simulink model "smMarsRover"  (R2024b)
settings: Solver=VariableStepAuto  StartTime=0.0  StopTime=51  RelTol=1e-3
PreLoadFcn:
  | run_sm
values from neighbouring files (symbols this model uses):
  arm_q0 = [-2.3554 -125.9144   49.8193 -175.7336  177.6446  180.0000]    [sm_mars_rover_params.m]
  goal_loc = [roverPath.x(end) roverPath.y(end)]    [sm_mars_rover_params.m]
  Z = fillmissing(Z, 'linear')    [setup.m]
undefined symbols (not defined in the file or in its folder): cameraData, Chassis_L, Chassis_width, eeConfig, Kd, Kd_arm, Kd_steer, Ki, Ki_arm, Ki_steer, Kp, Kp_arm, Kp_steer, Link1, Link2, Link3, R_disc_Link1, rover_accel, roverPath, t1, TrqLoLimit, TrqUpLimit, Wheel1_G, Wheel2_G, Wheel3_G, Wheel4_G, Wheel5_G, Wheel6_G, Wheel_Radius, X, Y
libraries: sm_lib x216, nesl_utility x51, slpidlib x3, simulink x3, robotcorelib x1, robotalgslib x1, simulink_extras x1
(part 7 of 7)

== system smMarsRover/RoverMotionControl&Planning/Rover /Wheels/RBWheel ==
  InnerWheel : sm_lib/Body Elements/File Solid  ExtGeomFileName=sm_mars_RoverData\mobility_wheel_inner.stl  UnitType=Custom  ExtGeomFileUnits=cm  StepReaderType=HEX  ExportConvexHullGeometry=off  InertiaType=Custom  BasedOnType=Density  Density=1000  DensityUnits=kg/m^3  Mass=0  MassUnits=kg  CenterOfMass=[0 0 0]  CenterOfMassUnits=m  MomentsOfInertia=[1 1 1]*0  MomentsOfInertiaUnits=kg*m^2  ProductsOfInertia=[0 0 0]  ProductsOfInertiaUnits=kg*m^2  GraphicType=FromGeometry  MarkerShape=Sphere  MarkerSize=10  GraphicVisPropType=AdvancedVisualProperties  GraphicDiffuseColor=[1.0 1.0 1.0]  GraphicOpacity=1.0  GraphicSpecularColor=[1 1 1 1.0]  GraphicAmbientColor=[0.15 0.15 0.15 1.0]  GraphicEmissiveColor=[0.1 0.1 0 1.0]  GraphicShininess=90  DoExposeReferenceFrame=on  SerializedFrames=<Frames/>
  OuterWheel : sm_lib/Body Elements/File Solid  ExtGeomFileName=sm_mars_RoverData\mobility_wheel_outer.stl  UnitType=Custom  ExtGeomFileUnits=cm  StepReaderType=HEX  ExportConvexHullGeometry=off  InertiaType=CalculateFromGeometry  BasedOnType=Density  Density=2700  DensityUnits=kg/m^3  Mass=1  MassUnits=kg  CenterOfMass=[0 0 0]  CenterOfMassUnits=m  MomentsOfInertia=[1 1 1]  MomentsOfInertiaUnits=kg*m^2  ProductsOfInertia=[0 0 0]  ProductsOfInertiaUnits=kg*m^2  GraphicType=FromGeometry  MarkerShape=Sphere  MarkerSize=10  GraphicVisPropType=AdvancedVisualProperties  GraphicDiffuseColor=[0.15 0.15 0.15]  GraphicOpacity=1.0  GraphicSpecularColor=[1 1 1 1.0]  GraphicAmbientColor=[0.15 0.15 0.15 1.0]  GraphicEmissiveColor=[0. 0. 0. 1]  GraphicShininess=100  DoExposeReferenceFrame=on  SerializedFrames=<Frames/>
  Point Cloud : sm_lib/Curves and Surfaces/Point Cloud  CoordinatesMatrix=new_wheel_points  CoordinatesMatrixUnits=cm  GraphicType=MarkerCloud  GraphicSphereRadius=0.25  GraphicSphereRadiusUnits=cm  GraphicVisPropType=SimpleVisualProperties  GraphicDiffuseColor=[1 0 0]  GraphicOpacity=1.0  GraphicSpecularColor=[0.5 0.5 0.5 1.0]  GraphicAmbientColor=[0.15 0.15 0.15 1.0]  GraphicEmissiveColor=[0.0 0.0 0.0 1.0]  GraphicShininess=75
  Rigid Transform : sm_lib/Frames and Transforms/Rigid Transform  RotationMethod=RotationMatrix  FollAlignAxisA=+X  BaseAlignAxisA=+Y  FollAlignAxisB=+Y  BaseAlignAxisB=+Z  RotationStandardAxis=+Z  RotationAngle=0.0  RotationAngleUnits=deg  RotationArbitraryAxis=[0 0 1]  RotationSequenceAxes=FollowerAxes  RotationSequence=XYX  RotationSequenceAngles=[0 0 0]  RotationSequenceAnglesUnits=deg  RotationMatrix=Wheel.WRJ_R  Quaternion=[1 0 0 0]  TranslationMethod=Cartesian  TranslationCartesianOffset=Wheel.WRJ_T  TranslationCartesianOffsetUnits=m  TranslationStandardAxis=+Z  TranslationStandardOffset=0  TranslationStandardOffsetUnits=m  TranslationROffset=0  TranslationROffsetUnits=m  TranslationThetaOffset=0  TranslationThetaOffsetUnits=deg  TranslationZOffset=0  TranslationZOffsetUnits=m
  Rigid Transform6 : sm_lib/Frames and Transforms/Rigid Transform  RotationMethod=StandardAxis  FollAlignAxisA=+X  BaseAlignAxisA=+Y  FollAlignAxisB=+Y  BaseAlignAxisB=+Z  RotationStandardAxis=+X  RotationAngle=90  RotationAngleUnits=deg  RotationArbitraryAxis=[0 0 1]  RotationSequenceAxes=FollowerAxes  RotationSequence=XYX  RotationSequenceAngles=[0 0 0]  RotationSequenceAnglesUnits=deg  RotationMatrix=[1 0 0; 0 1 0; 0 0 1]  Quaternion=[1 0 0 0]  TranslationMethod=None  TranslationCartesianOffset=[0 0 0]  TranslationCartesianOffsetUnits=cm  TranslationStandardAxis=+Y  TranslationStandardOffset=25.500/2  TranslationStandardOffsetUnits=cm  TranslationROffset=0  TranslationROffsetUnits=m  TranslationThetaOffset=0  TranslationThetaOffsetUnits=deg  TranslationZOffset=0  TranslationZOffsetUnits=m
  WRJ : PMIOPort  Side=Right
  G : PMIOPort  Port=2  Side=Left
  connections:
  Rigid Transform6/RConn1 -- WRJ/RConn1 -- Rigid Transform/RConn1
  OuterWheel/RConn1 -- Point Cloud/LConn1 -- Rigid Transform6/LConn1
  G/RConn1 -- Point Cloud/RConn1
  InnerWheel/RConn1 -- Rigid Transform/LConn1

== system smMarsRover/RoverMotionControl&Planning/Rover /Wheels/RFWheel ==
  InnerWheel : sm_lib/Body Elements/File Solid  ExtGeomFileName=sm_mars_RoverData\mobility_wheel_inner.stl  UnitType=Custom  ExtGeomFileUnits=cm  StepReaderType=HEX  ExportConvexHullGeometry=off  InertiaType=Custom  BasedOnType=Density  Density=1000  DensityUnits=kg/m^3  Mass=0  MassUnits=kg  CenterOfMass=[0 0 0]  CenterOfMassUnits=m  MomentsOfInertia=[1 1 1]*0  MomentsOfInertiaUnits=kg*m^2  ProductsOfInertia=[0 0 0]  ProductsOfInertiaUnits=kg*m^2  GraphicType=FromGeometry  MarkerShape=Sphere  MarkerSize=10  GraphicVisPropType=AdvancedVisualProperties  GraphicDiffuseColor=[1.0 1.0 1.0]  GraphicOpacity=1.0  GraphicSpecularColor=[1 1 1 1.0]  GraphicAmbientColor=[0.15 0.15 0.15 1.0]  GraphicEmissiveColor=[0.1 0.1 0 1.0]  GraphicShininess=90  DoExposeReferenceFrame=on  SerializedFrames=<Frames/>
  OuterWheel : sm_lib/Body Elements/File Solid  ExtGeomFileName=sm_mars_RoverData\mobility_wheel_outer.stl  UnitType=Custom  ExtGeomFileUnits=cm  StepReaderType=HEX  ExportConvexHullGeometry=off  InertiaType=CalculateFromGeometry  BasedOnType=Density  Density=2700  DensityUnits=kg/m^3  Mass=1  MassUnits=kg  CenterOfMass=[0 0 0]  CenterOfMassUnits=m  MomentsOfInertia=[1 1 1]  MomentsOfInertiaUnits=kg*m^2  ProductsOfInertia=[0 0 0]  ProductsOfInertiaUnits=kg*m^2  GraphicType=FromGeometry  MarkerShape=Sphere  MarkerSize=10  GraphicVisPropType=AdvancedVisualProperties  GraphicDiffuseColor=[0.15 0.15 0.15]  GraphicOpacity=1.0  GraphicSpecularColor=[1 1 1 1.0]  GraphicAmbientColor=[0.15 0.15 0.15 1.0]  GraphicEmissiveColor=[0. 0. 0. 1]  GraphicShininess=100  DoExposeReferenceFrame=on  SerializedFrames=<Frames/>
  Point Cloud : sm_lib/Curves and Surfaces/Point Cloud  CoordinatesMatrix=new_wheel_points  CoordinatesMatrixUnits=cm  GraphicType=MarkerCloud  GraphicSphereRadius=0.25  GraphicSphereRadiusUnits=cm  GraphicVisPropType=SimpleVisualProperties  GraphicDiffuseColor=[1 0 0]  GraphicOpacity=1.0  GraphicSpecularColor=[0.5 0.5 0.5 1.0]  GraphicAmbientColor=[0.15 0.15 0.15 1.0]  GraphicEmissiveColor=[0.0 0.0 0.0 1.0]  GraphicShininess=75
  Rigid Transform : sm_lib/Frames and Transforms/Rigid Transform  RotationMethod=RotationMatrix  FollAlignAxisA=+X  BaseAlignAxisA=+Y  FollAlignAxisB=+Y  BaseAlignAxisB=+Z  RotationStandardAxis=+Z  RotationAngle=0.0  RotationAngleUnits=deg  RotationArbitraryAxis=[0 0 1]  RotationSequenceAxes=FollowerAxes  RotationSequence=XYX  RotationSequenceAngles=[0 0 0]  RotationSequenceAnglesUnits=deg  RotationMatrix=Wheel.WRJ_R  Quaternion=[1 0 0 0]  TranslationMethod=Cartesian  TranslationCartesianOffset=Wheel.WRJ_T  TranslationCartesianOffsetUnits=m  TranslationStandardAxis=+Z  TranslationStandardOffset=0  TranslationStandardOffsetUnits=m  TranslationROffset=0  TranslationROffsetUnits=m  TranslationThetaOffset=0  TranslationThetaOffsetUnits=deg  TranslationZOffset=0  TranslationZOffsetUnits=m
  Rigid Transform6 : sm_lib/Frames and Transforms/Rigid Transform  RotationMethod=StandardAxis  FollAlignAxisA=+X  BaseAlignAxisA=+Y  FollAlignAxisB=+Y  BaseAlignAxisB=+Z  RotationStandardAxis=+X  RotationAngle=90  RotationAngleUnits=deg  RotationArbitraryAxis=[0 0 1]  RotationSequenceAxes=FollowerAxes  RotationSequence=XYX  RotationSequenceAngles=[0 0 0]  RotationSequenceAnglesUnits=deg  RotationMatrix=[1 0 0; 0 1 0; 0 0 1]  Quaternion=[1 0 0 0]  TranslationMethod=None  TranslationCartesianOffset=[0 0 0]  TranslationCartesianOffsetUnits=cm  TranslationStandardAxis=+Y  TranslationStandardOffset=25.500/2  TranslationStandardOffsetUnits=cm  TranslationROffset=0  TranslationROffsetUnits=m  TranslationThetaOffset=0  TranslationThetaOffsetUnits=deg  TranslationZOffset=0  TranslationZOffsetUnits=m
  WRJ : PMIOPort  Side=Right
  G : PMIOPort  Port=2  Side=Left
  connections:
  InnerWheel/RConn1 -- Rigid Transform/LConn1
  G/RConn1 -- Point Cloud/RConn1
  Rigid Transform6/LConn1 -- Point Cloud/LConn1 -- OuterWheel/RConn1
  Rigid Transform/RConn1 -- WRJ/RConn1 -- Rigid Transform6/RConn1

== system smMarsRover/RoverMotionControl&Planning/Rover /Wheels/RMWheel ==
  InnerWheel : sm_lib/Body Elements/File Solid  ExtGeomFileName=sm_mars_RoverData\mobility_wheel_inner.stl  UnitType=Custom  ExtGeomFileUnits=cm  StepReaderType=HEX  ExportConvexHullGeometry=off  InertiaType=Custom  BasedOnType=Density  Density=1000  DensityUnits=kg/m^3  Mass=0  MassUnits=kg  CenterOfMass=[0 0 0]  CenterOfMassUnits=m  MomentsOfInertia=[1 1 1]*0  MomentsOfInertiaUnits=kg*m^2  ProductsOfInertia=[0 0 0]  ProductsOfInertiaUnits=kg*m^2  GraphicType=FromGeometry  MarkerShape=Sphere  MarkerSize=10  GraphicVisPropType=AdvancedVisualProperties  GraphicDiffuseColor=[1.0 1.0 1.0]  GraphicOpacity=1.0  GraphicSpecularColor=[1 1 1 1.0]  GraphicAmbientColor=[0.15 0.15 0.15 1.0]  GraphicEmissiveColor=[0.1 0.1 0 1.0]  GraphicShininess=90  DoExposeReferenceFrame=on  SerializedFrames=<Frames/>
  OuterWheel : sm_lib/Body Elements/File Solid  ExtGeomFileName=sm_mars_RoverData\mobility_wheel_outer.stl  UnitType=Custom  ExtGeomFileUnits=cm  StepReaderType=HEX  ExportConvexHullGeometry=off  InertiaType=CalculateFromGeometry  BasedOnType=Density  Density=2700  DensityUnits=kg/m^3  Mass=1  MassUnits=kg  CenterOfMass=[0 0 0]  CenterOfMassUnits=m  MomentsOfInertia=[1 1 1]  MomentsOfInertiaUnits=kg*m^2  ProductsOfInertia=[0 0 0]  ProductsOfInertiaUnits=kg*m^2  GraphicType=FromGeometry  MarkerShape=Sphere  MarkerSize=10  GraphicVisPropType=AdvancedVisualProperties  GraphicDiffuseColor=[0.15 0.15 0.15]  GraphicOpacity=1.0  GraphicSpecularColor=[1 1 1 1.0]  GraphicAmbientColor=[0.15 0.15 0.15 1.0]  GraphicEmissiveColor=[0. 0. 0. 1]  GraphicShininess=100  DoExposeReferenceFrame=on  SerializedFrames=<Frames/>
  Point Cloud : sm_lib/Curves and Surfaces/Point Cloud  CoordinatesMatrix=new_wheel_points  CoordinatesMatrixUnits=cm  GraphicType=MarkerCloud  GraphicSphereRadius=0.25  GraphicSphereRadiusUnits=cm  GraphicVisPropType=SimpleVisualProperties  GraphicDiffuseColor=[1 0 0]  GraphicOpacity=1.0  GraphicSpecularColor=[0.5 0.5 0.5 1.0]  GraphicAmbientColor=[0.15 0.15 0.15 1.0]  GraphicEmissiveColor=[0.0 0.0 0.0 1.0]  GraphicShininess=75
  Rigid Transform : sm_lib/Frames and Transforms/Rigid Transform  RotationMethod=RotationMatrix  FollAlignAxisA=+X  BaseAlignAxisA=+Y  FollAlignAxisB=+Y  BaseAlignAxisB=+Z  RotationStandardAxis=+Z  RotationAngle=0.0  RotationAngleUnits=deg  RotationArbitraryAxis=[0 0 1]  RotationSequenceAxes=FollowerAxes  RotationSequence=XYX  RotationSequenceAngles=[0 0 0]  RotationSequenceAnglesUnits=deg  RotationMatrix=Wheel.WRJ_R  Quaternion=[1 0 0 0]  TranslationMethod=Cartesian  TranslationCartesianOffset=Wheel.WRJ_T  TranslationCartesianOffsetUnits=m  TranslationStandardAxis=+Z  TranslationStandardOffset=0  TranslationStandardOffsetUnits=m  TranslationROffset=0  TranslationROffsetUnits=m  TranslationThetaOffset=0  TranslationThetaOffsetUnits=deg  TranslationZOffset=0  TranslationZOffsetUnits=m
  Rigid Transform6 : sm_lib/Frames and Transforms/Rigid Transform  RotationMethod=StandardAxis  FollAlignAxisA=+X  BaseAlignAxisA=+Y  FollAlignAxisB=+Y  BaseAlignAxisB=+Z  RotationStandardAxis=+X  RotationAngle=90  RotationAngleUnits=deg  RotationArbitraryAxis=[0 0 1]  RotationSequenceAxes=FollowerAxes  RotationSequence=XYX  RotationSequenceAngles=[0 0 0]  RotationSequenceAnglesUnits=deg  RotationMatrix=[1 0 0; 0 1 0; 0 0 1]  Quaternion=[1 0 0 0]  TranslationMethod=None  TranslationCartesianOffset=[0 0 0]  TranslationCartesianOffsetUnits=cm  TranslationStandardAxis=+Y  TranslationStandardOffset=25.500/2  TranslationStandardOffsetUnits=cm  TranslationROffset=0  TranslationROffsetUnits=m  TranslationThetaOffset=0  TranslationThetaOffsetUnits=deg  TranslationZOffset=0  TranslationZOffsetUnits=m
  WRJ : PMIOPort  Side=Right
  G : PMIOPort  Port=2  Side=Left
  connections:
  InnerWheel/RConn1 -- Rigid Transform/LConn1
  G/RConn1 -- Point Cloud/RConn1
  Rigid Transform6/LConn1 -- Point Cloud/LConn1 -- OuterWheel/RConn1
  Rigid Transform/RConn1 -- WRJ/RConn1 -- Rigid Transform6/RConn1

== system smMarsRover/RoverMotionControl&Planning/Rover /Wheels/SteeringBracketLB  ==
  File Solid5 : sm_lib/Body Elements/File Solid  ExtGeomFileName=sm_mars_RoverData\mobility_steering_bracket.stl  UnitType=Custom  ExtGeomFileUnits=cm  StepReaderType=HEX  ExportConvexHullGeometry=off  InertiaType=CalculateFromGeometry  BasedOnType=Density  Density=1000  DensityUnits=kg/m^3  Mass=0  MassUnits=kg  CenterOfMass=[0 0 0]  CenterOfMassUnits=m  MomentsOfInertia=[1 1 1]*0  MomentsOfInertiaUnits=kg*m^2  ProductsOfInertia=[0 0 0]  ProductsOfInertiaUnits=kg*m^2  GraphicType=FromGeometry  MarkerShape=Sphere  MarkerSize=10  GraphicVisPropType=AdvancedVisualProperties  GraphicDiffuseColor=[0.2 0.2 0.2]  GraphicOpacity=1.0  GraphicSpecularColor=[1 1 1 1.0]  GraphicAmbientColor=[0.15 0.15 0.15 1.0]  GraphicEmissiveColor=[0.0 0.0 0.0 1.0]  GraphicShininess=90  DoExposeReferenceFrame=on  SerializedFrames=<Frames/>
  Reference Frame : sm_lib/Frames and Transforms/Reference Frame
  Rigid Transform : sm_lib/Frames and Transforms/Rigid Transform  RotationMethod=RotationMatrix  FollAlignAxisA=+X  BaseAlignAxisA=+Y  FollAlignAxisB=+Y  BaseAlignAxisB=+Z  RotationStandardAxis=+Z  RotationAngle=0.0  RotationAngleUnits=deg  RotationArbitraryAxis=[0 0 1]  RotationSequenceAxes=FollowerAxes  RotationSequence=XYX  RotationSequenceAngles=[0 0 0]  RotationSequenceAnglesUnits=deg  RotationMatrix=SB.SRJ_R  Quaternion=[1 0 0 0]  TranslationMethod=Cartesian  TranslationCartesianOffset=SB.SRJ_T  TranslationCartesianOffsetUnits=m  TranslationStandardAxis=+Z  TranslationStandardOffset=0  TranslationStandardOffsetUnits=m  TranslationROffset=0  TranslationROffsetUnits=m  TranslationThetaOffset=0  TranslationThetaOffsetUnits=deg  TranslationZOffset=0  TranslationZOffsetUnits=m
  Rigid Transform1 : sm_lib/Frames and Transforms/Rigid Transform  RotationMethod=RotationMatrix  FollAlignAxisA=+X  BaseAlignAxisA=+Y  FollAlignAxisB=+Y  BaseAlignAxisB=+Z  RotationStandardAxis=+Z  RotationAngle=0.0  RotationAngleUnits=deg  RotationArbitraryAxis=[0 0 1]  RotationSequenceAxes=FollowerAxes  RotationSequence=XYX  RotationSequenceAngles=[0 0 0]  RotationSequenceAnglesUnits=deg  RotationMatrix=SB.WRJ_R  Quaternion=[1 0 0 0]  TranslationMethod=Cartesian  TranslationCartesianOffset=SB.WRJ_T  TranslationCartesianOffsetUnits=m  TranslationStandardAxis=+Z  TranslationStandardOffset=0  TranslationStandardOffsetUnits=m  TranslationROffset=0  TranslationROffsetUnits=m  TranslationThetaOffset=0  TranslationThetaOffsetUnits=deg  TranslationZOffset=0  TranslationZOffsetUnits=m
  SRJ : PMIOPort  Side=Left
  WRJ : PMIOPort  Port=2  Side=Right
  connections:
  Rigid Transform/RConn1 -- SRJ/RConn1
  WRJ/RConn1 -- Rigid Transform1/RConn1
  Reference Frame/RConn1 -- Rigid Transform1/LConn1 -- Rigid Transform/LConn1 -- File Solid5/RConn1

== system smMarsRover/RoverMotionControl&Planning/Rover /Wheels/SteeringBracketLF ==
  File Solid5 : sm_lib/Body Elements/File Solid  ExtGeomFileName=sm_mars_RoverData\mobility_steering_bracket.stl  UnitType=Custom  ExtGeomFileUnits=cm  StepReaderType=HEX  ExportConvexHullGeometry=off  InertiaType=CalculateFromGeometry  BasedOnType=Density  Density=1000  DensityUnits=kg/m^3  Mass=0  MassUnits=kg  CenterOfMass=[0 0 0]  CenterOfMassUnits=m  MomentsOfInertia=[1 1 1]*0  MomentsOfInertiaUnits=kg*m^2  ProductsOfInertia=[0 0 0]  ProductsOfInertiaUnits=kg*m^2  GraphicType=FromGeometry  MarkerShape=Sphere  MarkerSize=10  GraphicVisPropType=AdvancedVisualProperties  GraphicDiffuseColor=[0.2 0.2 0.2]  GraphicOpacity=1.0  GraphicSpecularColor=[1 1 1 1.0]  GraphicAmbientColor=[0.15 0.15 0.15 1.0]  GraphicEmissiveColor=[0.0 0.0 0.0 1.0]  GraphicShininess=90  DoExposeReferenceFrame=on  SerializedFrames=<Frames/>
  Reference Frame : sm_lib/Frames and Transforms/Reference Frame
  Rigid Transform : sm_lib/Frames and Transforms/Rigid Transform  RotationMethod=RotationMatrix  FollAlignAxisA=+X  BaseAlignAxisA=+Y  FollAlignAxisB=+Y  BaseAlignAxisB=+Z  RotationStandardAxis=+Z  RotationAngle=0.0  RotationAngleUnits=deg  RotationArbitraryAxis=[0 0 1]  RotationSequenceAxes=FollowerAxes  RotationSequence=XYX  RotationSequenceAngles=[0 0 0]  RotationSequenceAnglesUnits=deg  RotationMatrix=SB.SRJ_R  Quaternion=[1 0 0 0]  TranslationMethod=Cartesian  TranslationCartesianOffset=SB.SRJ_T  TranslationCartesianOffsetUnits=m  TranslationStandardAxis=+Z  TranslationStandardOffset=0  TranslationStandardOffsetUnits=m  TranslationROffset=0  TranslationROffsetUnits=m  TranslationThetaOffset=0  TranslationThetaOffsetUnits=deg  TranslationZOffset=0  TranslationZOffsetUnits=m
  Rigid Transform1 : sm_lib/Frames and Transforms/Rigid Transform  RotationMethod=RotationMatrix  FollAlignAxisA=+X  BaseAlignAxisA=+Y  FollAlignAxisB=+Y  BaseAlignAxisB=+Z  RotationStandardAxis=+Z  RotationAngle=0.0  RotationAngleUnits=deg  RotationArbitraryAxis=[0 0 1]  RotationSequenceAxes=FollowerAxes  RotationSequence=XYX  RotationSequenceAngles=[0 0 0]  RotationSequenceAnglesUnits=deg  RotationMatrix=SB.WRJ_R  Quaternion=[1 0 0 0]  TranslationMethod=Cartesian  TranslationCartesianOffset=SB.WRJ_T  TranslationCartesianOffsetUnits=m  TranslationStandardAxis=+Z  TranslationStandardOffset=0  TranslationStandardOffsetUnits=m  TranslationROffset=0  TranslationROffsetUnits=m  TranslationThetaOffset=0  TranslationThetaOffsetUnits=deg  TranslationZOffset=0  TranslationZOffsetUnits=m
  SRJ : PMIOPort  Side=Left
  WRJ : PMIOPort  Port=2  Side=Right
  connections:
  Rigid Transform/RConn1 -- SRJ/RConn1
  WRJ/RConn1 -- Rigid Transform1/RConn1
  File Solid5/RConn1 -- Reference Frame/RConn1 -- Rigid Transform1/LConn1 -- Rigid Transform/LConn1

== system smMarsRover/RoverMotionControl&Planning/Rover /Wheels/SteeringBracketRB ==
  File Solid5 : sm_lib/Body Elements/File Solid  ExtGeomFileName=sm_mars_RoverData\mobility_steering_bracket.stl  UnitType=Custom  ExtGeomFileUnits=cm  StepReaderType=HEX  ExportConvexHullGeometry=off  InertiaType=CalculateFromGeometry  BasedOnType=Density  Density=1000  DensityUnits=kg/m^3  Mass=0  MassUnits=kg  CenterOfMass=[0 0 0]  CenterOfMassUnits=m  MomentsOfInertia=[1 1 1]*0  MomentsOfInertiaUnits=kg*m^2  ProductsOfInertia=[0 0 0]  ProductsOfInertiaUnits=kg*m^2  GraphicType=FromGeometry  MarkerShape=Sphere  MarkerSize=10  GraphicVisPropType=AdvancedVisualProperties  GraphicDiffuseColor=[0.2 0.2 0.2]  GraphicOpacity=1.0  GraphicSpecularColor=[1 1 1 1.0]  GraphicAmbientColor=[0.15 0.15 0.15 1.0]  GraphicEmissiveColor=[0.0 0.0 0.0 1.0]  GraphicShininess=90  DoExposeReferenceFrame=on  SerializedFrames=<Frames/>
  Reference Frame : sm_lib/Frames and Transforms/Reference Frame
  Rigid Transform : sm_lib/Frames and Transforms/Rigid Transform  RotationMethod=RotationMatrix  FollAlignAxisA=+X  BaseAlignAxisA=+Y  FollAlignAxisB=+Y  BaseAlignAxisB=+Z  RotationStandardAxis=+Z  RotationAngle=0.0  RotationAngleUnits=deg  RotationArbitraryAxis=[0 0 1]  RotationSequenceAxes=FollowerAxes  RotationSequence=XYX  RotationSequenceAngles=[0 0 0]  RotationSequenceAnglesUnits=deg  RotationMatrix=SB.SRJ_R  Quaternion=[1 0 0 0]  TranslationMethod=Cartesian  TranslationCartesianOffset=SB.SRJ_T  TranslationCartesianOffsetUnits=m  TranslationStandardAxis=+Z  TranslationStandardOffset=0  TranslationStandardOffsetUnits=m  TranslationROffset=0  TranslationROffsetUnits=m  TranslationThetaOffset=0  TranslationThetaOffsetUnits=deg  TranslationZOffset=0  TranslationZOffsetUnits=m
  Rigid Transform1 : sm_lib/Frames and Transforms/Rigid Transform  RotationMethod=RotationMatrix  FollAlignAxisA=+X  BaseAlignAxisA=+Y  FollAlignAxisB=+Y  BaseAlignAxisB=+Z  RotationStandardAxis=+Z  RotationAngle=0.0  RotationAngleUnits=deg  RotationArbitraryAxis=[0 0 1]  RotationSequenceAxes=FollowerAxes  RotationSequence=XYX  RotationSequenceAngles=[0 0 0]  RotationSequenceAnglesUnits=deg  RotationMatrix=SB.WRJ_R  Quaternion=[1 0 0 0]  TranslationMethod=Cartesian  TranslationCartesianOffset=SB.WRJ_T  TranslationCartesianOffsetUnits=m  TranslationStandardAxis=+Z  TranslationStandardOffset=0  TranslationStandardOffsetUnits=m  TranslationROffset=0  TranslationROffsetUnits=m  TranslationThetaOffset=0  TranslationThetaOffsetUnits=deg  TranslationZOffset=0  TranslationZOffsetUnits=m
  SRJ : PMIOPort  Side=Left
  WRJ : PMIOPort  Port=2  Side=Right
  connections:
  Rigid Transform/LConn1 -- Rigid Transform1/LConn1 -- Reference Frame/RConn1 -- File Solid5/RConn1
  WRJ/RConn1 -- Rigid Transform1/RConn1
  Rigid Transform/RConn1 -- SRJ/RConn1

== system smMarsRover/RoverMotionControl&Planning/Rover /Wheels/SteeringBracketRF ==
  File Solid5 : sm_lib/Body Elements/File Solid  ExtGeomFileName=sm_mars_RoverData\mobility_steering_bracket.stl  UnitType=Custom  ExtGeomFileUnits=cm  StepReaderType=HEX  ExportConvexHullGeometry=off  InertiaType=CalculateFromGeometry  BasedOnType=Density  Density=1000  DensityUnits=kg/m^3  Mass=0  MassUnits=kg  CenterOfMass=[0 0 0]  CenterOfMassUnits=m  MomentsOfInertia=[1 1 1]*0  MomentsOfInertiaUnits=kg*m^2  ProductsOfInertia=[0 0 0]  ProductsOfInertiaUnits=kg*m^2  GraphicType=FromGeometry  MarkerShape=Sphere  MarkerSize=10  GraphicVisPropType=AdvancedVisualProperties  GraphicDiffuseColor=[0.2 0.2 0.2]  GraphicOpacity=1.0  GraphicSpecularColor=[1 1 1 1.0]  GraphicAmbientColor=[0.15 0.15 0.15 1.0]  GraphicEmissiveColor=[0.0 0.0 0.0 1.0]  GraphicShininess=90  DoExposeReferenceFrame=on  SerializedFrames=<Frames/>
  Reference Frame : sm_lib/Frames and Transforms/Reference Frame
  Rigid Transform : sm_lib/Frames and Transforms/Rigid Transform  RotationMethod=RotationMatrix  FollAlignAxisA=+X  BaseAlignAxisA=+Y  FollAlignAxisB=+Y  BaseAlignAxisB=+Z  RotationStandardAxis=+Z  RotationAngle=0.0  RotationAngleUnits=deg  RotationArbitraryAxis=[0 0 1]  RotationSequenceAxes=FollowerAxes  RotationSequence=XYX  RotationSequenceAngles=[0 0 0]  RotationSequenceAnglesUnits=deg  RotationMatrix=SB.SRJ_R  Quaternion=[1 0 0 0]  TranslationMethod=Cartesian  TranslationCartesianOffset=SB.SRJ_T  TranslationCartesianOffsetUnits=m  TranslationStandardAxis=+Z  TranslationStandardOffset=0  TranslationStandardOffsetUnits=m  TranslationROffset=0  TranslationROffsetUnits=m  TranslationThetaOffset=0  TranslationThetaOffsetUnits=deg  TranslationZOffset=0  TranslationZOffsetUnits=m
  Rigid Transform1 : sm_lib/Frames and Transforms/Rigid Transform  RotationMethod=RotationMatrix  FollAlignAxisA=+X  BaseAlignAxisA=+Y  FollAlignAxisB=+Y  BaseAlignAxisB=+Z  RotationStandardAxis=+Z  RotationAngle=0.0  RotationAngleUnits=deg  RotationArbitraryAxis=[0 0 1]  RotationSequenceAxes=FollowerAxes  RotationSequence=XYX  RotationSequenceAngles=[0 0 0]  RotationSequenceAnglesUnits=deg  RotationMatrix=SB.WRJ_R  Quaternion=[1 0 0 0]  TranslationMethod=Cartesian  TranslationCartesianOffset=SB.WRJ_T  TranslationCartesianOffsetUnits=m  TranslationStandardAxis=+Z  TranslationStandardOffset=0  TranslationStandardOffsetUnits=m  TranslationROffset=0  TranslationROffsetUnits=m  TranslationThetaOffset=0  TranslationThetaOffsetUnits=deg  TranslationZOffset=0  TranslationZOffsetUnits=m
  SRJ : PMIOPort  Side=Left
  WRJ : PMIOPort  Port=2  Side=Right
  connections:
  Rigid Transform/RConn1 -- SRJ/RConn1
  WRJ/RConn1 -- Rigid Transform1/RConn1
  File Solid5/RConn1 -- Reference Frame/RConn1 -- Rigid Transform1/LConn1 -- Rigid Transform/LConn1

== system smMarsRover/RoverMotionControl&Planning/Rover Path Planning And Control/hold/RoverStopTime ==
  Enable : Inport
  Clock : Clock
  Constant2 : Constant
  Display : Display
  Enabled Subsystem1 : Subsystem  TreatAsAtomicUnit=on
      settings: MinAlgLoopOccurrences=on
  Switch : Switch  Criteria=u2 > Threshold  SaturateOnIntegerOverflow=off  InputSameDT=off
  Unit Delay : UnitDelay  SampleTime=-1  HasFrameUpgradeWarning=on
  DeAccelTime : Outport
  wires:
  Enabled Subsystem1/1(Out1) -> Switch/2
  Enable/1 -> Enabled Subsystem1/Enable
  Switch/1 -> Unit Delay/1
  Unit Delay/1 -> Display/1, DeAccelTime/1, Switch/1
  Clock/1 -> Switch/3
  Constant2/1 -> Enabled Subsystem1/1(In1)

== system smMarsRover/RoverMotionControl&Planning/Rover Path Planning And Control/hold/RoverStopTime/Enabled Subsystem1 ==
  In1 : Inport
  Enable : EnablePort
  Out1 : Outport
  wires:
  In1/1 -> Out1/1

== matlab function smMarsRover/RoverMotionControl&Planning/Rover Path Planning And Control/Ackerman Steer Angle/Ackerman Steering Angle Formulation ==
  data: delta input; LFsteerAng output; L input; RFsteerAng output; d input; R output; L_R output; R_R output
function [LFsteerAng,RFsteerAng,R,L_R,R_R] = fcn(delta,L,d)
% Function to compute ackerman steering angles from a bicycle steer angle.

R = L/tand(abs(delta));

if delta < 0
    LFsteerAng = atan2d(L,(R+d/2));
    RFsteerAng = atan2d(L,(R-d/2));
    L_R = (R+d/2);
    R_R = (R-d/2);
else
    LFsteerAng = -atan2d(L,(R-d/2));
    RFsteerAng = -atan2d(L,(R+d/2));
    L_R = (R-d/2);
    R_R = (R+d/2);
end

end

== matlab function smMarsRover/RoverMotionControl&Planning/Rover Path Planning And Control/Chassis Velocity To Wheel Speed ==
  data: desChassisSpeed input; wheel_speed_LF output; wheel_r input; steer_ang input; wheel_speed_LM output; wheel_speed_LB output; R input; L input; L_R input; R_R input; wheel_speed_RF output; wheel_speed_RM output; wheel_speed_RB output
function [wheel_speed_LF,wheel_speed_LM,wheel_speed_LB,...
    wheel_speed_RF,wheel_speed_RM,wheel_speed_RB] = fcn(desChassisSpeed,wheel_r,steer_ang,R,L,L_R,R_R)
% Function to compute wheel speed from a desired linear velocity and
% desired path.

if any(abs(steer_ang) > 0)

    wheel_speed_LF = (desChassisSpeed/wheel_r)*sqrt(L_R^2 + L^2)/R;
    wheel_speed_LM = desChassisSpeed * L_R/(R*wheel_r);
    wheel_speed_LB = (desChassisSpeed/wheel_r)*sqrt(L_R^2 + L^2)/R;
    wheel_speed_RF = -(desChassisSpeed/wheel_r)*sqrt(R_R^2 + L^2)/R;
    wheel_speed_RM = -desChassisSpeed * R_R/(R*wheel_r);
    wheel_speed_RB = -(desChassisSpeed/wheel_r)*sqrt(R_R^2 + L^2)/R;

else
    wheel_speed_LF = desChassisSpeed / wheel_r;
    wheel_speed_LM = desChassisSpeed / wheel_r;
    wheel_speed_LB = desChassisSpeed / wheel_r;
    wheel_speed_RF = -desChassisSpeed / wheel_r;
    wheel_speed_RM = -desChassisSpeed / wheel_r;
    wheel_speed_RB = -desChassisSpeed / wheel_r;
end

end

== matlab function smMarsRover/Manipulator Plant Model And Control/ Trajectory Planner/Planner Subsystem/Task Scheduler ==
  settings: updateMethod=DISCRETE
  data: wayPts output; reset_t output; samplePickCmd output; sampleDropCmd output; actJointAngles input; desJointAngles input; samplePickSense input; sampleDropSense input; currentTime input; stop output
function [wayPts,reset_t,samplePickCmd,sampleDropCmd,stop]  = fcn(actJointAngles,desJointAngles,samplePickSense,sampleDropSense,currentTime)
% This function plans the top level tasks for the arm. The end effector goal
% and sample interaction joint configuration modes depend on the current task mode.
%
% mode 0: home/initial position (waypt 1) (samplePickCmd Off)
% mode 1-2: move to the position close the sample (waypt 3 via waypt 2) (samplePickCmd Off)
% mode 3-4 : move to sample position and pick up sample (waypt 4) (samplePickCmd On)
% mode 5 : move back to the position close the sample (waypt 3) (samplePickCmd On)
% mode 6 : move to the position close to the sample storage unit (waypt 5) (samplePickCmd On)
% mode 7-8 : move to sample storage position and drop/collect sample (waypt 6) (sampleDropCmd On)
% mode 9 : move back to the position close to the sample storage unit (samplePickCmd,sampleDropCmd On)
% mode 10-11 :move to home position 

maxErrPos = 0.5;
actJointAngles =actJointAngles';
persistent mode resetTime
stop = 0;
if isempty(mode)
    mode = 0;
    resetTime = 0;
end

reset_t =  resetTime;

switch mode

    case 0
        % Home Position
        wayPts = [desJointAngles(1,:);desJointAngles(1,:)];
        samplePickCmd = false;
        sampleDropCmd = false;

        if all(abs(actJointAngles-desJointAngles(1,:)) < maxErrPos)
            resetTime = currentTime;
            if sampleDropSense == 1
                mode = 0;
            else
                mode = 1;
            end
        end

    case 1
        
        wayPts = desJointAngles(1:2,:);
        samplePickCmd = false;
        sampleDropCmd = false;

        if all(abs(actJointAngles-desJointAngles(2,:)) < maxErrPos)
            resetTime = currentTime;
            mode = 2;
        end

    case 2
        % Move to the position close the sample
        wayPts = desJointAngles(2:3,:);
        samplePickCmd = false;
        sampleDropCmd = false;

        if all(abs(actJointAngles-desJointAngles(3,:)) < maxErrPos)
            resetTime = currentTime;
            mode = 3;
        end

    case 3
        % Move to sample position
        wayPts = desJointAngles(3:4,:);
        samplePickCmd = false;
        sampleDropCmd = false;

        if all(abs(actJointAngles-desJointAngles(4,:)) < maxErrPos)
            resetTime = currentTime;
            mode = 4;
        end

    case 4
        % Stay at sample position and pick up the sample
        wayPts = [desJointAngles(4,:); desJointAngles(4,:)];
        samplePickCmd = true;
        sampleDropCmd = false;

        if all(abs(actJointAngles-desJointAngles(4,:)) < maxErrPos) && samplePickSense == 1
            resetTime = currentTime;
            mode = 5;
        end

    case 5
        % Move back to the position close to the sample
        wayPts = desJointAngles(4:-1:3,:);
        samplePickCmd = true;
        sampleDropCmd = false;

        if all(abs(actJointAngles-desJointAngles(3,:)) < maxErrPos)
            resetTime = currentTime;
            mode = 6;
        end


    case 6
        % Move the position close to the sample storage unit
        wayPts = [desJointAngles(3,:) ;desJointAngles(5,:)];
        samplePickCmd = true;
        sampleDropCmd = false;

        if all(abs(actJointAngles-desJointAngles(5,:)) < maxErrPos)
            resetTime = currentTime;
            mode = 7;
        end

    case 7
        % Move to the sample storage unit position
        wayPts = desJointAngles(5:6,:);
        sampleDropCmd = false;
        samplePickCmd = true;

        if all(abs(actJointAngles-desJointAngles(6,:)) < maxErrPos)
            resetTime = currentTime;
            mode = 8;
        end

    case 8
        % Stay at sample drop position, drop and collect the sample
        wayPts = [desJointAngles(6,:);desJointAngles(6,:)];

        sampleDropCmd = true;
        samplePickCmd = true;

        if (all(abs(actJointAngles-desJointAngles(6,:)) < maxErrPos)) && sampleDropSense == 1
            resetTime = currentTime;
            mode = 9;
        end

    case 9
        % Move back to the position close to the sample storage unit
        wayPts = desJointAngles(6:-1:5,:);
        sampleDropCmd = true;
        samplePickCmd = true;

        if all(abs(actJointAngles-desJointAngles(5,:)) < maxErrPos)
            resetTime = currentTime;
            mode = 10;
        end

    case 10
        % Move to home position via waypt 2
        wayPts = [desJointAngles(5,:); desJointAngles(7,:)];
        sampleDropCmd = true;
        samplePickCmd = true;

        if all(abs(actJointAngles-desJointAngles(7,:)) < maxErrPos)
            resetTime = currentTime;
            mode = 11;
        end

    case 11
        % Move to home position
        wayPts = [desJointAngles(7,:); desJointAngles(1,:)];
        sampleDropCmd = true;
        samplePickCmd = true;

        if all(abs(actJointAngles-desJointAngles(1,:)) < maxErrPos)
            resetTime = currentTime;           
            mode = 12;
        end
   
    case 12
        % Mission Complete
        wayPts = [desJointAngles(7,:); desJointAngles(1,:)];
        sampleDropCmd = true;
        samplePickCmd = true;
        mode = 12;
        stop = 1;
    otherwise
        error('invalid mode');

end

end

== matlab function smMarsRover/Manipulator Plant Model And Control/ Trajectory Planner/Planner Subsystem/Inverse Kinematics ==
  data: jointSpaceWayPts output; eePoseDes input; eeIgs input; samplePosition input; prevWayPts input
function  jointSpaceWayPts = fcn(eePoseDes,eeIgs,samplePosition,prevWayPts)
% Wrapper around sm_mars_rover_arm_ik.m
% Takes end effector targets and initial guesses and returns all the
% actuator positions corresponding to each target.

coder.extrinsic("sm_mars_rover_arm_ik");

jointSpaceWayPts = zeros(7,6); %#ok<PREALL> 

% End effector Targets and initial guesses derived from sample location
samplePose = [samplePosition 175 0 91];
sample_position_eef = samplePose;
sample_position_eef_ig = [90.0000 -200.0000   90.0000   40.0000  170.0000  -10.0000];%[90   -200  160  90 170 -60];
sample_pos_init_eef = [sample_position_eef(1) sample_position_eef(2) sample_position_eef(3)+0.1 sample_position_eef(4) sample_position_eef(5) sample_position_eef(6)];
sample_pos_init_eef_ig = [90.0000 -200.0000   90.0000   40.0000  170.0000  -10.0000];%[90   -200  160  90 170 0];

% Combine precomputed end effector targets (waypts 1,2,5,6) with the
% ones derived from sample location (waypts 3,4) to create a set of
% task space waypoints for planning the trajectory.

EndEffTargets = ... 
    [eePoseDes(1,:);...% Waypt 1,(HomePos)
     eePoseDes(2,:);...% Waypt 2
    sample_pos_init_eef;...% Waypt 3,(Position near sample)
    sample_position_eef;...% Waypt 4 (Sample position)
    eePoseDes(3,:);... % Waypt 5,(Position near storage unit)
    eePoseDes(4,:);...% Waypt 6,(Sample storage position)
    eePoseDes(5,:);...
    ];

EndEffIgs = ...
     [eeIgs(1,:);...
     eeIgs(2,:);...
     sample_pos_init_eef_ig ;...  
     sample_position_eef_ig;...
     eeIgs(3,:);...
     eeIgs(4,:);...
     eeIgs(5,:);...
    ];

% Obtain joint space waypoints by calling IK for each end effector target
if prevWayPts == zeros(7,6)
[jointSpaceWayPts,solvedFlag] =  sm_mars_rover_arm_ik(EndEffTargets,EndEffIgs); %#ok<ASGLU> 
else
jointSpaceWayPts = prevWayPts;
end

end

== matlab function smMarsRover/RoverMotionControl&Planning/Rover Path Planning And Control/Target Dir To Bicycle Steer Angle/Rad2Deg ==
  data: u input; y output
function y = fcn(u)
y = rad2deg(u);

== matlab function smMarsRover/Rover Outputs/CalcSpeed ==
  data: u input; y output
function y = fcn(u)
y = sqrt(u(1)^2 + u(2)^2);
end

== matlab function smMarsRover/RoverMotionControl&Planning/Rover Pose Sensing/theta_act ==
  data: u input; z output; y output; x output
function [z,y,x] = fcn(u)
out = rotm2eul(u);
z = out(1);
y = out(2);
x = out(3);
end

== matlab function smMarsRover/RoverMotionControl&Planning/Rover Pose Sensing/CalcSpeed ==
  data: u input; y output
function y = fcn(u)
y = sqrt(u(1)^2 + u(2)^2);
end

== matlab function smMarsRover/Manipulator Plant Model And Control/Rover Arm/rad2deg ==
  data: u input; y output
function y = fcn(u)

y = rad2deg(u);

== matlab function smMarsRover/Manipulator Plant Model And Control/ Trajectory Planner/SamplePickUpCmdLogic/DistanceError ==
  data: u input; flag output
function flag  = fcn(u)

distanceErr = sqrt(u(1)^2 + u(2)^2 +u(3)^2);

if distanceErr < 1e-2
    flag = true;
else
flag = false;
end

end

== matlab function smMarsRover/Manipulator Plant Model And Control/ Trajectory Planner/SampleDropOffCmdLogic/DistanceError ==
  data: u input; flag output
function flag  = fcn(u)

distanceErr = sqrt(u(1)^2 + u(2)^2 +u(3)^2);

if distanceErr < 1e-2
    flag = true;
else
flag = false;
end

end

== matlab function smMarsRover/RoverMotionControl&Planning/Rover Path Planning And Control/Trapezoidal Vel Profile ==
  data: linVel input; t input; t1 input; lin_Vel_out output; accel input; deaccelStartTime input
function lin_Vel_out = fcn(linVel,t,t1,accel,deaccelStartTime)
% Function to create a trapezoidal profile for rover's desired linear
% velocity

t2 = linVel/accel + t1;
t3 = deaccelStartTime + 0.2;
tf = linVel/accel + t3;

if t>=t1 && t<t2 
    lin_Vel_out = accel*(t-t1);

elseif t>=t2 && t < t3 
    lin_Vel_out = linVel;

elseif t>= t3 && t < tf 
    lin_Vel_out = linVel-accel*(t-t3);

else
    lin_Vel_out = 0;    
end


end
